simulink model "Hardware_Integration"  (R2016a)
settings: Solver=FixedStepAuto  StartTime=0.0  StopTime=inf  FixedStep=0.01  RelTol=1e-3
undefined symbols (not defined in the file): sigbuilder_block
libraries: arduinolib x11, simulink x4, arduinosensorlib x1
settings Model: SimulationMode=external  ExtModeTrigDuration=2  Creator=mmb94  LastModifiedBy=mmb94
settings DataIOCC: ReturnWorkspaceOutputs=on
settings OptimizationCC: EnhancedBackFolding=on  PassReuseOutputArgsAs=Individual arguments  OptimizeModelRefInitCode=on  MaxStackSize=64
settings DebuggingCC: ParameterTunabilityLossMsg=error  SFUnexpectedBacktrackingDiag=error  SFNoUnconditionalDefaultTransitionDiag=error
settings HardwareCC: ProdBitPerInt=16  ProdBitPerPointer=16  ProdLargestAtomicFloat=None  ProdWordSize=8  ProdHWDeviceType=Atmel->AVR
settings SFSimCC: SimUseLocalCustomCode=on
settings RTWCC: SystemTargetFile=ert.tlc  HardwareBoard=Arduino Mega 2560  TLCOptions=-aInlineSetEventsForThisBaseRateFcn=TLC_FALSE -aSuppressMultiTaskScheduler=TLC_FALSE -aRateBasedStepFcn=1  TemplateMakefile=ert_default_tmf  GenerateReport=on  RTWUseLocalCustomCode=on  Toolchain=Arduino AVR  BuildConfiguration=Faster Runs  IncludeHyperlinkInReport=on  LaunchReport=on  GenerateTraceInfo=on  GenerateTraceReport=on  GenerateTraceReportSl=on  GenerateTraceReportSf=on  GenerateTraceReportEml=on
settings CodeAppCC: ForceParamTrailComments=on  IgnoreCustomStorageClasses=off  OperatorAnnotations=on  SimulinkDataObjDesc=on  SFDataObjDesc=on  InsertBlockDesc=on
settings ERTTargetCC: MultiwordLength=256  SupportContinuousTime=on  SupportVariableSizeSignals=on  ExtModeStaticAllocSize=2048
settings ConfigComp: CovMetricSettings=dwe  CovHtmlReporting=off  CovSaveCumulativeToWorkspaceVar=off  CovSaveSingleToWorkspaceVar=off  CovExternalEMLEnable=on

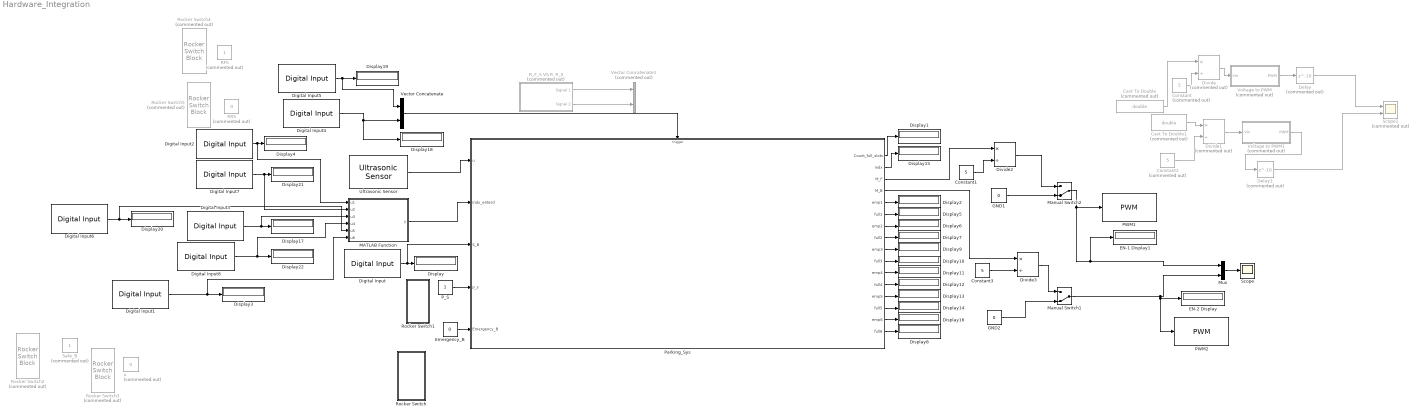
== system Hardware_Integration ==
  " PWM1" : arduinolib/PWM  pinNumber=5  EnableInputFrequency=off  InitialFrequency=2000  InitialDutyCycle=0  NotificationType=None  blockPlatform=arduino
  " PWM2" : arduinolib/PWM  pinNumber=6  EnableInputFrequency=off  InitialFrequency=2000  InitialDutyCycle=0  NotificationType=None  blockPlatform=arduino
  Cast To Double : DataTypeConversion  Commented=on  OutDataTypeStr=double
  Cast To Double1 : DataTypeConversion  Commented=on  OutDataTypeStr=double
  Constant : Constant  Commented=on  Value=5
  Constant1 : Constant  Value=5
  Constant2 : Constant  Commented=on  Value=5
  Constant3 : Constant  Value=5
  Delay : Delay  Commented=on  DelayLength=10
  Delay1 : Delay  Commented=on  DelayLength=10
  Digital Input : arduinolib/Digital Input  pinNumber=52  sampleTime=0.1  blockPlatform=arduino
  Digital Input1 : arduinolib/Digital Input  pinNumber=50  sampleTime=0.1  blockPlatform=arduino
  Digital Input2 : arduinolib/Digital Input  pinNumber=48  sampleTime=0.1  blockPlatform=arduino
  Digital Input3 : arduinolib/Digital Input  pinNumber=46  sampleTime=0.1  blockPlatform=arduino
  Digital Input4 : arduinolib/Digital Input  pinNumber=53  sampleTime=0.1  blockPlatform=arduino
  Digital Input5 : arduinolib/Digital Input  pinNumber=51  sampleTime=0.1  blockPlatform=arduino
  Digital Input6 : arduinolib/Digital Input  pinNumber=49  sampleTime=0.1  blockPlatform=arduino
  Digital Input7 : arduinolib/Digital Input  pinNumber=47  sampleTime=0.1  blockPlatform=arduino
  Digital Input8 : arduinolib/Digital Input  pinNumber=45  sampleTime=0.1  blockPlatform=arduino
  Display{,1..22} (23 alike) : Display
  Divide : Product  Commented=on  Inputs=*/
  Divide1 : Product  Commented=on  Inputs=*/
  Divide2 : Product  Inputs=*/
  Divide3 : Product  Inputs=*/
  EN-1 Display1 : Display
  EN-2 Display : Display
  Emergency_B : Constant  Value=0
  GND1 : Constant  Value=0
  GND2 : Constant  Value=0
  MATLAB Function : MATLAB Function  TreatAsAtomicUnit=on
  Manual Switch1 : ManualSwitch  CurrentSetting=0
  Manual Switch2 : ManualSwitch  CurrentSetting=0
  Mux : Mux  Inputs=2
  P_S : Constant
  Parking_Sys : Stateflow chart  TreatAsAtomicUnit=on
  RFS : Constant  Commented=on
  RRS : Constant  Commented=on  Value=0
  R_F_S VS R_R_S : Subsystem  Tag=STV Subsys  Commented=on  LoadFcn=sigbuilder_block('load');  StartFcn=sigbuilder_block('start');  StopFcn=sigbuilder_block('stop');  ClipboardFcn=sigbuilder_block('clipboard');  mask(Sigbuilder block){}
      mask help: Simulink:masks:SigbuilderBlock_MD
      mask init:
      | if ~strcmp(get_param(bdroot(gcbh),'SimulationStatus'),'stopped') tuvar = sigbuilder_block('maskInit'); end
      settings: CopyFcn=sigbuilder_block('copy');  DeleteFcn=sigbuilder_block('delete');  ModelCloseFcn=sigbuilder_block('modelClose');  PreSaveFcn=sigbuilder_block('preSave');  PauseFcn=sigbuilder_block('pause');  ContinueFcn=sigbuilder_block('continue');  NameChangeFcn=sigbuilder_block('namechange');  OpenFcn=sigbuilder_block('open',[6 30 1012.5 447.75 ]);  CloseFcn=sigbuilder_block('close');
      mask Display: plot(0, 0, 100, 100,[2, 2, 32, 32, 2], [68, 8, 8, 68, 68],[32, 2], [38, 38], [32, 19, 2],[53, 60, 44], [32, 17, 17, 2],[16, 16, 31, 31]);txt = getActiveGroup(gcbh);text(2, 100, txt,'verticalAlignment', 'top');
  Rocker Switch : Subsystem  DialogController=hmiCreateDDGDialog  IsWebBlock=on  mask(MWDashboardBlock){webBlockId=faa10a22-7694-454d-90cf-b69878c71df5, webBlockType=rockerswitch, ShowInLibBrowser=on, ShowInitialText=on, HMISrcModelName=state_chart_final}
      mask prompts: webBlockId "WebBlock Id"; webBlockType "WebBlock Type"; HMISrcModelName "Source Model"
      mask help: Set on/off value to tune parameters or variables.
      mask Help: helpview([docroot '/mapfiles/simulink.map'], 'hmi_switch')
      mask Display:
      | if strcmp(get_param(bdroot(gcb),'BlockDiagramType'),'library')
      |  image([(matlabroot) '/toolbox/simulink/hmi/icons/RockerSwitch.png'])
      | end
  Rocker Switch1 : Subsystem  DialogController=hmiCreateDDGDialog  IsWebBlock=on  mask(MWDashboardBlock){webBlockId=f7060ea5-3ad6-45d0-b3c9-e244c4784b3f, webBlockType=rockerswitch, ShowInLibBrowser=on, ShowInitialText=on, HMISrcModelName=state_chart_final}
      mask prompts: webBlockId "WebBlock Id"; webBlockType "WebBlock Type"; HMISrcModelName "Source Model"
      mask help: Set on/off value to tune parameters or variables.
      mask Help: helpview([docroot '/mapfiles/simulink.map'], 'hmi_switch')
      mask Display:
      | if strcmp(get_param(bdroot(gcb),'BlockDiagramType'),'library')
      |  image([(matlabroot) '/toolbox/simulink/hmi/icons/RockerSwitch.png'])
      | end
  Rocker Switch{2..5} (4 alike) : RockerSwitchBlock  Commented=on
      settings: Values={{'Off', 'On'}, [0 1]}
  Safe_B : Constant  Commented=on
  Scope : Scope
  Scope1 : Scope  Commented=on  NumInputPorts=2
  Ultrasonic Sensor : arduinosensorlib/Ultrasonic Sensor  NumSignalPins=2  TrigPin=7  EchoPin=8  SignalPin=3  SampleTime_=0.1  blockPlatform=ARDUINO
  Vector Concatenate : Concatenate
  Vector Concatenate1 : Concatenate  Commented=on
  Voltage to PWM : Subsystem  Commented=on
  Voltage to PWM1 : Subsystem  Commented=on
  u : Constant  Commented=on  Value=0
  wires:
  Parking_Sys/2(indx) -> Display15/1
  R_F_S VS R_R_S/1(Signal 1) -> Vector Concatenate1/1
  R_F_S VS R_R_S/2(Signal 2) -> Vector Concatenate1/2
  Vector Concatenate/1 -> Parking_Sys/Trigger
  Parking_Sys/6(full1) -> Display5/1
  Parking_Sys/7(emp2) -> Display6/1
  Parking_Sys/16(full6) -> Display8/1
  Parking_Sys/8(full2) -> Display7/1
  Parking_Sys/5(emp1) -> Display2/1
  Parking_Sys/9(emp3) -> Display9/1
  Parking_Sys/10(full3) -> Display10/1
  Parking_Sys/11(emp4) -> Display11/1
  Parking_Sys/12(full4) -> Display12/1
  Parking_Sys/13(emp5) -> Display13/1
  Parking_Sys/14(full5) -> Display14/1
  Parking_Sys/15(emp6) -> Display16/1
  Parking_Sys/1(Count_full_slots) -> Display1/1
  Voltage to PWM/1(PWM) -> Delay/1
  Divide/1 -> Voltage to PWM/1(VIn)
  Cast To Double/1 -> Divide/1
  Constant/1 -> Divide/2
  Constant2/1 -> Divide1/2
  Cast To Double1/1 -> Divide1/1
  Divide1/1 -> Voltage to PWM1/1(VIn)
  Delay/1 -> Scope1/1
  Voltage to PWM1/1(PWM) -> Delay1/1
  Delay1/1 -> Scope1/2
  Ultrasonic Sensor/1 -> Parking_Sys/1(u)
  Digital Input6/1 -> MATLAB Function/5(u5), Display20/1
  Digital Input7/1 -> Display21/1, MATLAB Function/2(u2)
  Digital Input1/1 -> Display3/1, MATLAB Function/6(u6)
  Digital Input3/1 -> Display17/1, MATLAB Function/3(u3)
  Digital Input8/1 -> MATLAB Function/4(u4), Display22/1
  Digital Input2/1 -> MATLAB Function/1(u1), Display4/1
  Digital Input4/1 -> Vector Concatenate/2, Display18/1
  MATLAB Function/1(y) -> Parking_Sys/2(indx_enterd)
  Digital Input5/1 -> Vector Concatenate/1, Display19/1
  Digital Input/1 -> Parking_Sys/3(S_B), Display/1
  Emergency_B/1 -> Parking_Sys/5(Emergency_B)
  P_S/1 -> Parking_Sys/4(p_s)
  Constant3/1 -> Divide3/2
  Divide3/1 -> Manual Switch1/1
  Constant1/1 -> Divide2/2
  Manual Switch1/1 -> " PWM2"/1, EN-2 Display/1, Mux/2
  Mux/1 -> Scope/1
  Manual Switch2/1 -> Mux/1, EN-1 Display1/1, " PWM1"/1
  GND2/1 -> Manual Switch1/2
  Parking_Sys/4(M_B) -> Divide3/1
  Parking_Sys/3(M_F) -> Divide2/1
  Divide2/1 -> Manual Switch2/1
  GND1/1 -> Manual Switch2/2

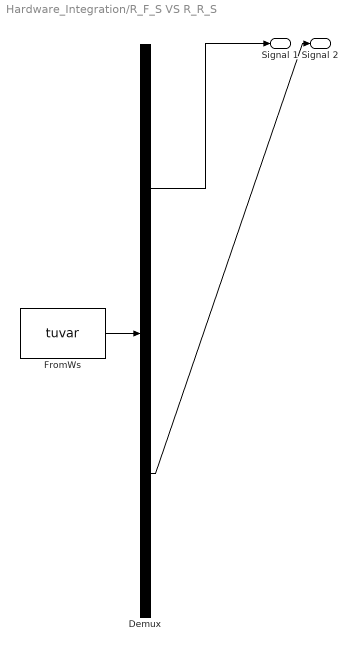
== system Hardware_Integration/R_F_S VS R_R_S ==
  Demux : Demux  Tag=STV Demux  Outputs=2
  FromWs : FromWorkspace  Tag=STV FromWs  VariableName=tuvar  SampleTime=0
      SigBuilderData=|
      | common.afterFinalStr = 'Extrapolate'
      | common.sampleTime = 0
      | dataSet.timeRange = [0 10]
      | dataSet.name = 'Group 1'
      | sbobj.Groups.Name = 'Group 1'
      | sbobj.Groups.Signals(1).Name = 'Signal 1'
      | sbobj.Groups.Signals(1).XData = [0 2.01 2.01 9.01 9.01 10]
      | sbobj.Groups.Signals(1).YData = [0 0 1 1 0 0]
      | sbobj.Groups.Signals(2).Name = 'Signal 2'
      | sbobj.Groups.Signals(2).XData = [0 5 10]
      | sbobj.Groups.Signals(2).YData = [0 0 0]
  Signal 1 : Outport  Tag=STV Outport
  Signal 2 : Outport  Tag=STV Outport  Port=2
  wires:
  Demux/1 -> Signal 1/1
  FromWs/1 -> Demux/1
  Demux/2 -> Signal 2/1

== system Hardware_Integration/Rocker Switch ==

== system Hardware_Integration/Rocker Switch1 ==

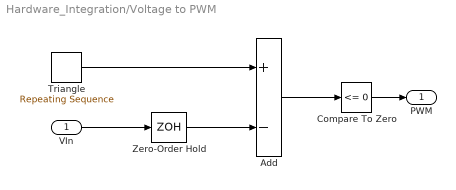
== system Hardware_Integration/Voltage to PWM ==
  VIn : Inport
  Add : Sum  Inputs=+-  SampleTime=1/10000
  Compare To Zero : simulink/Logic and Bit Operations/Compare To Zero  relop=<=  OutDataTypeStr=uint8
  Triangle : simulink/Sources/Repeating Sequence  rep_seq_t=[0 1/100/4 3/100/4 1/100]  rep_seq_y=[0.5 0 1 0.5]
  Zero-Order Hold : ZeroOrderHold  SampleTime=1/10000
  PWM : Outport
  wires:
  Triangle/1 -> Add/1
  VIn/1 -> Zero-Order Hold/1
  Add/1 -> Compare To Zero/1
  Compare To Zero/1 -> PWM/1
  Zero-Order Hold/1 -> Add/2

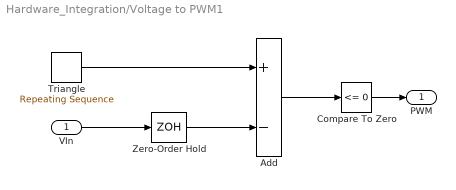
== system Hardware_Integration/Voltage to PWM1 ==
  VIn : Inport
  Add : Sum  Inputs=+-  SampleTime=1/10000
  Compare To Zero : simulink/Logic and Bit Operations/Compare To Zero  relop=<=  OutDataTypeStr=uint8
  Triangle : simulink/Sources/Repeating Sequence  rep_seq_t=[0 1/100/4 3/100/4 1/100]  rep_seq_y=[0.5 0 1 0.5]
  Zero-Order Hold : ZeroOrderHold  SampleTime=1/10000
  PWM : Outport
  wires:
  Zero-Order Hold/1 -> Add/2
  Compare To Zero/1 -> PWM/1
  Add/1 -> Compare To Zero/1
  VIn/1 -> Zero-Order Hold/1
  Triangle/1 -> Add/1

== matlab function Hardware_Integration/MATLAB Function ==
  data: u1 input; y output; u2 input; u3 input; u4 input; u5 input; u6 input
function y = fcn(u1,u2,u3,u4,u5,u6)
if (u1==1)
y=1;
end
if(u2==1)
y=2;
end
if(u3==1)
y=3;
end
if(u4==1)
y=4;
end
if(u5==1)
y=5;
end
if(u6==1)
y=6;
end

== stateflow chart Hardware_Integration/Parking_Sys ==
  state System
    state Power_on
      state Slots [parallel]
        entry: emp1 = 1;
        entry:emp2 = 1;
        entry:emp3 = 1;
        entry:emp4 = 1;
        entry:emp5 = 1;
        entry:emp6 = 1;
        entry: full1 = 0;
        entry: full2=0;
        entry: full3=0;
        entry: full4=0;
        entry: full5=0;
        entry: full6=0;
        settings: executionOrder=1
        (history)
        state Slot1
          entry: indx =1;
          state check
          state Full
            entry: full1 = 1;
            entry: M_F=0;
            entry: M_B=0;
          state Empty
            entry: emp1 = 1;
            entry: M_F=0;
            entry: M_B=0;
          (default) -> System.Power_on.Slots.Slot1.check
          System.Power_on.Slots.Slot1.check -> System.Power_on.Slots.Slot1.Full [order 2] : [full1==1&&emp1==0]
          System.Power_on.Slots.Slot1.check -> System.Power_on.Slots.Slot1.Empty [order 1] : [emp1==1&& full1==0]
          System.Power_on.Slots.Slot1.Empty -> System.Power_on.Slots.Slot1.Full [order 1] : R_F_S[u == 0]{emp1=0;}
          System.Power_on.Slots.Slot1.Full -> System.Power_on.Slots.Slot1.Empty [order 1] : R_R_S[indx_enterd == indx && u==1]{full1=0;}
        state Slot6
          entry: indx =6;
          state check
          state Full
            entry: full6 = 1;
            entry: M_F=0;
            entry: M_B=0;
          state Empty
            entry: emp6 = 1;
            entry: M_F=0;
            entry: M_B=0;
          (default) -> System.Power_on.Slots.Slot6.check
          System.Power_on.Slots.Slot6.check -> System.Power_on.Slots.Slot6.Empty [order 2] : [emp6==1&& full6==0]
          System.Power_on.Slots.Slot6.check -> System.Power_on.Slots.Slot6.Full [order 1] : [full6==1&&emp6==0]
          System.Power_on.Slots.Slot6.Empty -> System.Power_on.Slots.Slot6.Full [order 1] : R_F_S[u == 0]{emp6=0;}
          System.Power_on.Slots.Slot6.Full -> System.Power_on.Slots.Slot6.Empty [order 3] : R_R_S[indx_enterd == indx && u==1]{full6=0;}
        state Slot2
          entry: indx =2;
          %entry: M_F=0;
          %entry: M_B=0;
          state check
          state Empty
            entry: emp2 = 1;
            entry: M_F=0;
            entry: M_B=0;
          state Full
            entry: full2 = 1;
            entry: M_F=0;
            entry: M_B=0;
          (default) -> System.Power_on.Slots.Slot2.check
          System.Power_on.Slots.Slot2.check -> System.Power_on.Slots.Slot2.Full [order 2] : [full2==1&&emp2==0]
          System.Power_on.Slots.Slot2.check -> System.Power_on.Slots.Slot2.Empty [order 1] : [emp2==1&& full2==0]
          System.Power_on.Slots.Slot2.Empty -> System.Power_on.Slots.Slot2.Full [order 1] : R_F_S[u==0]{emp2=0;}
          System.Power_on.Slots.Slot2.Full -> System.Power_on.Slots.Slot2.Empty [order 3] : R_R_S[indx_enterd==indx && u==1]{full2=0;}
        state Slot5
          entry: indx=5;
          state check
          state Empty
            entry: emp5 = 1;
            entry: M_F=0;
            entry: M_B=0;
          state Full
            entry: full5 = 1;
            entry: M_F=0;
            entry: M_B=0;
          (default) -> System.Power_on.Slots.Slot5.check
          System.Power_on.Slots.Slot5.check -> System.Power_on.Slots.Slot5.Full [order 2] : [full5==1&&emp5==0]
          System.Power_on.Slots.Slot5.check -> System.Power_on.Slots.Slot5.Empty [order 1] : [emp5==1&& full5==0]
          System.Power_on.Slots.Slot5.Empty -> System.Power_on.Slots.Slot5.Full [order 2] : R_F_S[u == 0]{emp5=0;}
          System.Power_on.Slots.Slot5.Full -> System.Power_on.Slots.Slot5.Empty [order 1] : R_R_S[indx_enterd == indx && u==1]{full5=0;}
        state Slot4
          entry: indx =4;
          state check
          state Empty
            entry: emp4 = 1;
            entry: M_F=0;
            entry: M_B=0;
          state Full
            entry: full4 = 1;
            entry: M_F=0;
            entry: M_B=0;
          (default) -> System.Power_on.Slots.Slot4.check
          System.Power_on.Slots.Slot4.check -> System.Power_on.Slots.Slot4.Empty [order 1] : [emp4==1&& full4==0]
          System.Power_on.Slots.Slot4.check -> System.Power_on.Slots.Slot4.Full [order 2] : [full4==1&&emp4==0]
          System.Power_on.Slots.Slot4.Empty -> System.Power_on.Slots.Slot4.Full [order 1] : R_F_S[u==0]{emp4=0;}
          System.Power_on.Slots.Slot4.Full -> System.Power_on.Slots.Slot4.Empty [order 1] : R_R_S[indx_enterd==indx && u==1]{full4=0;}
        state Slot3
          entry: indx =3;
          state check
          state Full
            entry: full3 = 1;
            entry: M_F=0;
            entry: M_B=0;
          state Empty
            entry: emp3 = 1;
            entry: M_F=0;
            entry: M_B=0;
          (default) -> System.Power_on.Slots.Slot3.check
          System.Power_on.Slots.Slot3.check -> System.Power_on.Slots.Slot3.Full [order 1] : [full3==1&&emp3==0]
          System.Power_on.Slots.Slot3.check -> System.Power_on.Slots.Slot3.Empty [order 2] : [emp3==1&& full3==0]
          System.Power_on.Slots.Slot3.Full -> System.Power_on.Slots.Slot3.Empty [order 1] : R_R_S[indx_enterd==indx && u==1]{full3=0;}
          System.Power_on.Slots.Slot3.Empty -> System.Power_on.Slots.Slot3.Full [order 1] : R_F_S[u==0]{emp3=0;}
        (default) -> Slot1
        System.Power_on.Slots.Slot6.Empty -> Slot1 [order 3] : R_R_S[indx_enterd ~= indx && (3<indx_enterd) &&(indx_enterd<indx) ]{M_B=1}
        System.Power_on.Slots.Slot1.Empty -> Slot6 [order 3] : R_R_S[indx_enterd ~= indx && (indx_enterd>3) ]{M_B=1}
        System.Power_on.Slots.Slot1.Full -> Slot6 [order 4] : R_F_S[(emp6==1 | emp5==1)&&( full2==1)&& S_B==1&& u==1 ]{M_B=1}
        System.Power_on.Slots.Slot1.Full -> Slot6 [order 5] : R_R_S[indx_enterd ~= indx && (indx_enterd>3) && u==1 ]{M_B=1}
        System.Power_on.Slots.Slot1.Full -> Slot2 [order 3] : R_F_S[(emp2==1 | emp3==1 | emp4==1) && S_B==1 && u==1]{M_F=1}
        System.Power_on.Slots.Slot1.Full -> Slot2 [order 2] : R_R_S[(indx_enterd ~=indx) && (indx<indx_enterd) && indx_enterd<=3 && u==1 ]{M_F=1}
        System.Power_on.Slots.Slot1.Empty -> Slot2 [order 2] : R_R_S[(indx_enterd ~=indx) && (indx<indx_enterd)&& (indx_enterd<=3) ]{M_F=1}
        System.Power_on.Slots.Slot6.Full -> Slot1 [order 1] : R_F_S[( emp1==1 | emp2==1 | emp3==1 )&& ( full5==1 )&& S_B ==1&& u==1 ]{M_B=1}
        System.Power_on.Slots.Slot6.Full -> Slot1 [order 2] : R_R_S[indx_enterd ~= indx && (3<indx_enterd)&&(indx_enterd<indx)&& u==1  ]{M_B=1}
        System.Power_on.Slots.Slot2.Empty -> Slot1 [order 2] : R_R_S[indx_enterd ~= indx && (indx_enterd<indx | indx_enterd>4) ]{M_B=1}
        System.Power_on.Slots.Slot2.Full -> Slot1 [order 1] : R_F_S[(emp1==1 | emp6==1)&&( full3==1) && S_B ==1 && u==1 ]{M_B=1}
        System.Power_on.Slots.Slot2.Full -> Slot1 [order 2] : R_R_S[indx_enterd ~= indx && (indx_enterd<indx | indx_enterd>4)&& u==1  ]{M_B=1}
        System.Power_on.Slots.Slot6.Full -> Slot5 [order 4] : R_F_S[(emp4==1 | emp5==1)&&( full1==1) && S_B ==1&& u==1 ]{M_B=1}
        System.Power_on.Slots.Slot6.Full -> Slot5 [order 5] : R_R_S[indx_enterd ~= indx && (indx_enterd<indx ) && u==1 ]{M_B=1}
        System.Power_on.Slots.Slot6.Empty -> Slot5 [order 2] : R_R_S[indx_enterd ~= indx && (indx_enterd<indx ) ]{M_B=1}
        System.Power_on.Slots.Slot5.Full -> Slot6 [order 5] : R_R_S[(indx_enterd ~=indx) &&( (indx<indx_enterd)| indx_enterd<3 )&& u==1 ]{M_F=1}
        System.Power_on.Slots.Slot5.Full -> Slot6 [order 4] : R_F_S[( emp6==1 | emp1==1 | emp2==1 )&&( full4==1 ) && S_B==1&& u==1 ]{M_F=1}
        System.Power_on.Slots.Slot5.Empty -> Slot6 [order 3] : R_R_S[(indx_enterd ~=indx) &&( (indx<indx_enterd)| indx_enterd<3 )]{M_F=1}
        System.Power_on.Slots.Slot2.Empty -> Slot3 [order 3] : R_R_S[(indx_enterd ~=indx) && (indx<indx_enterd<=3)]{M_F=1}
        System.Power_on.Slots.Slot2.Full -> Slot3 [order 4] : R_F_S[( emp3==1 | emp4==1 | emp5==1 )&&( full1==1) && S_B==1&& u==1 ]{M_F=1}
        System.Power_on.Slots.Slot2.Full -> Slot3 [order 5] : R_R_S[(indx_enterd ~=indx) && (indx<indx_enterd<=3) && u==1 ]{M_F=1}
        System.Power_on.Slots.Slot3.Empty -> Slot2 [order 2] : R_R_S[indx_enterd ~= indx && (indx_enterd<indx ) ]{M_B=1}
        System.Power_on.Slots.Slot3.Full -> Slot2 [order 2] : R_F_S[(emp1==1 | emp2==1)&&( full4==1)&& S_B ==1&& u==1 ]{M_B=1}
        System.Power_on.Slots.Slot3.Full -> Slot2 [order 3] : R_R_S[indx_enterd ~= indx && (indx_enterd<indx ) && u==1 ]{M_B=1}
        System.Power_on.Slots.Slot5.Full -> Slot4 [order 2] : R_F_S[(emp3==1 | emp4==1)&& (full6==1) && S_B ==1&& u==1 ]{M_B=1}
        System.Power_on.Slots.Slot5.Full -> Slot4 [order 3] : R_R_S[indx_enterd ~= indx && (indx_enterd<indx )&& u==1  ]{M_B=1}
        System.Power_on.Slots.Slot5.Empty -> Slot4 [order 1] : R_R_S[indx_enterd ~= indx && (indx_enterd<indx ) ]{M_B=1}
        System.Power_on.Slots.Slot4.Full -> Slot5 [order 5] : R_F_S[( emp5==1 | emp6==1| emp1==1 )&&( full3==1 ) && S_B==1&& u==1 ]{M_F=1}
        System.Power_on.Slots.Slot4.Full -> Slot5 [order 4] : R_R_S[(indx_enterd ~=indx) && (indx<indx_enterd)&& u==1 ]{M_F=1}
        System.Power_on.Slots.Slot4.Empty -> Slot5 [order 3] : R_R_S[(indx_enterd ~=indx) && (indx<indx_enterd)]{M_F=1}
        System.Power_on.Slots.Slot3.Empty -> Slot4 [order 3] : R_R_S[(indx_enterd ~=indx) && (indx<indx_enterd)]{M_F=1}
        System.Power_on.Slots.Slot4.Empty -> Slot3 [order 2] : R_R_S[indx_enterd ~= indx && (indx_enterd<indx ) ]{M_B=1}
        System.Power_on.Slots.Slot3.Full -> Slot4 [order 4] : R_F_S[(emp4==1 | emp5==1 | emp6==1)&&( full2==1 ) && S_B==1&& u==1 ]{M_F=1}
        System.Power_on.Slots.Slot3.Full -> Slot4 [order 5] : R_R_S[(indx_enterd ~=indx) && (indx<indx_enterd)&& u==1 ]{M_F=1}
        System.Power_on.Slots.Slot4.Full -> Slot3 [order 2] : R_F_S[(emp2==1 | emp3==1 )&&( full5==1)& S_B ==1&& u==1 ]{M_B=1}
        System.Power_on.Slots.Slot4.Full -> Slot3 [order 3] : R_R_S[indx_enterd ~= indx && (indx_enterd<indx )&& u==1  ]{M_B=1}
      state LCD [parallel]
        settings: executionOrder=2
        state Count_full_slot [parallel]
          during: Count_full_slots = full1+ full2 +full3+full4+full5+full6
          settings: executionOrder=1
    state Power_off1
      entry: M_F=0;
      entry: M_B=0;
    Power_off1 -> Power_on : [p_s ==1]
    Power_on -> Power_off1 : [p_s ==0]
    (default) -> Power_off1
  state Emergency_stop
    entry: M_F=0;
    entry: M_B=0;
    entry: Count_full_slots =-1;
  (default) -> System
  Emergency_stop -> System : [Emergency_B==0]
  System -> Emergency_stop : [Emergency_B==1]
  data: u input; indx_enterd input; S_B input; p_s input; Count_full_slots output; indx output; M_F output; M_B output; emp1 output; full1 output; Emergency_B input; emp2 output; full2 output; emp3 output; full3 output; emp4 output; full4 output; emp5 output; full5 output; emp6 output; full6 output
  events: R_F_S input RISING_EDGE_EVENT; R_R_S input RISING_EDGE_EVENT
